simulink model "link_flat"  (R2025b)
settings: Solver=FixedStepAuto  StartTime=0.0  StopTime=10.0  RelTol=1e-3
undefined symbols (not defined in the file): link_flat_params, Ts_inner
settings Model: DataDictionary=project.sldd  Creator=Nick  LastModifiedBy=Rakete

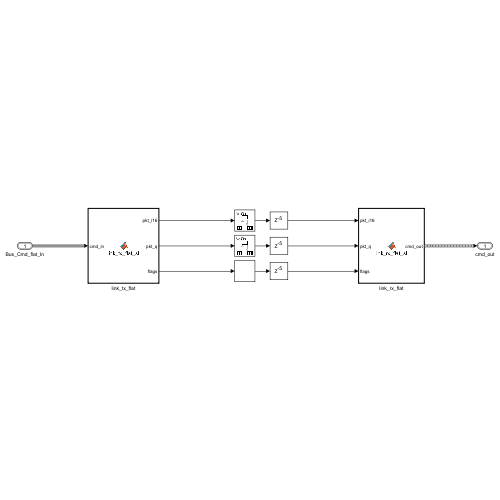
[thumbnail: Simulink's stored preview of the top-level diagram]
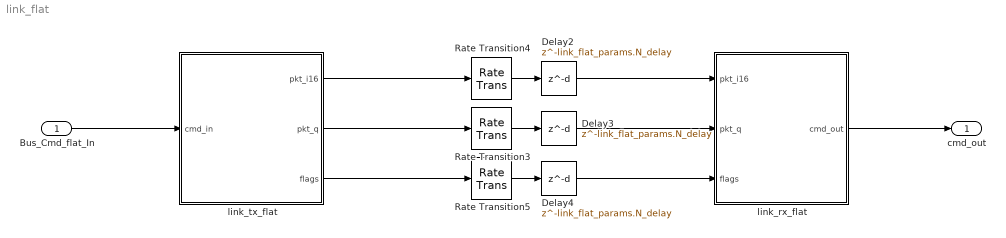
== system link_flat ==
  Bus_Cmd_flat_In : Inport  OutDataTypeStr=Bus: Bus_Cmd_flat
  Delay2 : Delay  DelayLength=link_flat_params.N_delay  InitialCondition=link_flat_params.pkt_init_delay  SampleTime=Ts_inner
  Delay3 : Delay  DelayLength=link_flat_params.N_delay  InitialCondition=link_flat_params.q_init_delay  SampleTime=Ts_inner
  Delay4 : Delay  DelayLength=link_flat_params.N_delay  InitialCondition=link_flat_params.flags_init_delay  SampleTime=Ts_inner
  Rate Transition3 : RateTransition  OutPortSampleTime=Ts_sim
  Rate Transition4 : RateTransition  OutPortSampleTime=Ts_sim
  Rate Transition5 : RateTransition  OutPortSampleTime=Ts_sim
  link_rx_flat : MATLAB Function  TreatAsAtomicUnit=on
  link_tx_flat : MATLAB Function  TreatAsAtomicUnit=on
  cmd_out : Outport  OutDataTypeStr=Bus: Bus_Cmd_flat
  wires:
  Rate Transition3/1 -> Delay3/1
  Rate Transition4/1 -> Delay2/1
  link_tx_flat/1(pkt_i16) -> Rate Transition4/1
  Delay2/1 -> link_rx_flat/1(pkt_i16)
  link_tx_flat/2(pkt_q) -> Rate Transition3/1
  Delay3/1 -> link_rx_flat/2(pkt_q)
  Rate Transition5/1 -> Delay4/1
  link_tx_flat/3(flags) -> Rate Transition5/1
  Delay4/1 -> link_rx_flat/3(flags)
  Bus_Cmd_flat_In/1 -> link_tx_flat/1(cmd_in)
  link_rx_flat/1(cmd_out) -> cmd_out/1

== matlab function link_flat/link_tx_flat ==
  data: cmd_in input Bus: Bus_Cmd_flat; pkt_i16 output int16 size=[13 1]; pkt_q output uint32 size=1; flags output size=[2 1]; link_flat_params parameter
function [pkt_i16, pkt_q, flags] = link_tx_flat_sl(cmd_in, link_flat_params)
%#codegen
% WRAPPER — code liegt in
% scripts\flatness\link_tx_flat.m - dieser Block ruft sie nur auf
[pkt_i16, pkt_q, flags] = link_tx_flat(cmd_in, link_flat_params);
end

== matlab function link_flat/link_rx_flat ==
  data: pkt_i16 input int16 size=[13 1]; cmd_out output Bus: Bus_Cmd_flat; pkt_q input uint32 size=1; flags input size=[2 1]; link_flat_params parameter
function cmd_out = link_rx_flat_sl(pkt_i16, pkt_q, flags, link_flat_params)
%#codegen
% WRAPPER — code liegt in
% scripts\flatness\link_rx_flat.m - dieser Block ruft sie nur auf
cmd_out = link_rx_flat(pkt_i16, pkt_q, flags, link_flat_params);
end
